simulink model "VS_CS_R4"  (R2018a)
settings: Solver=ode45  StartTime=0.0  StopTime=0.1  FixedStep=50e-6  RelTol=1e-9
libraries: fl_lib x12, nesl_utility x6
settings Model: Creator=mmi-vsa  LastModifiedBy=acs-mmi
settings DataIOCC: SaveFormat=Array
settings OptimizationCC: BlockReduction=off  BooleanDataType=off  LifeSpan=inf
settings DebuggingCC: SaveWithParameterizedLinksMsg=none  UnderspecifiedInitializationDetection=Classic  MergeDetectMultiDrivingBlocksExec=none  SignalResolutionControl=TryResolveAllWithWarning  SFUnexpectedBacktrackingDiag=warning  SFNoUnconditionalDefaultTransitionDiag=warning  SFExecutionAtInitializationDiag=none
settings HardwareCC: ProdBitPerPointer=32  ProdBitPerSizeT=32  ProdBitPerPtrDiffT=32  ProdLargestAtomicFloat=None  ProdIntDivRoundTo=Undefined  ProdEndianess=Unspecified  ProdWordSize=32  ProdHWDeviceType=32-bit Generic  TargetUnknown=on
settings ModelReferenceCC: PropagateSignalLabelsOutOfModel=off
settings CodeAppCC: StateflowObjectComments=on
settings GRTTargetCC: TargetLangStandard=C89/C90 (ANSI)  GeneratePreprocessorConditionals=Disable all
settings ConfigComp: CovMetricSettings=dw  CovHtmlReporting=on  CovSaveCumulativeToWorkspaceVar=on  CovSaveSingleToWorkspaceVar=on  CovExternalEMLEnable=off  CovSFcnEnable=off
settings SimscapeCC: SimscapeNormalizeSystem=off

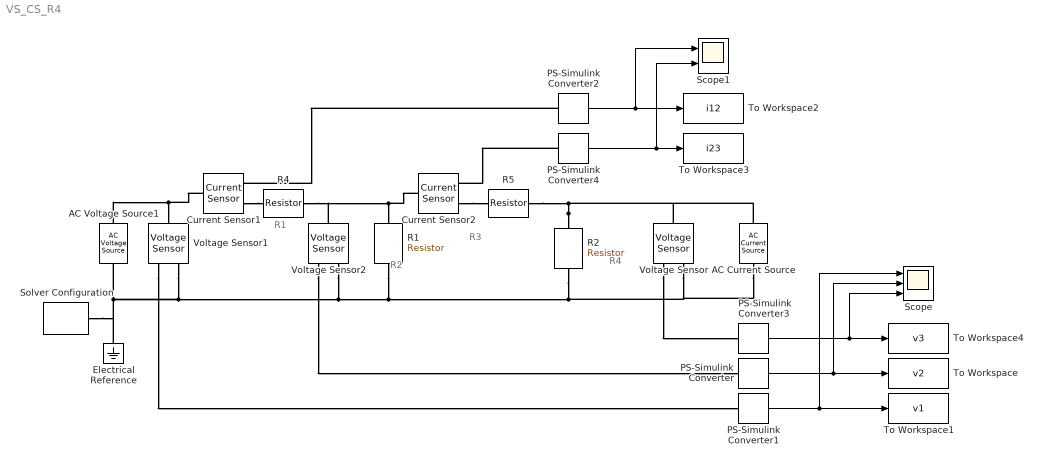
== system VS_CS_R4 ==
  note: R4
  note: R2
  note: R3
  note: R1
  AC Current Source : fl_lib/Electrical/Electrical Sources/AC Current Source  amp=1 A  shift=90 deg  frequency=50 Hz  omega=0 rad/s
      settings: SourceProductName=Simscape  SourceProductBaseCode=SS
  AC Voltage Source1 : fl_lib/Electrical/Electrical Sources/AC Voltage Source  amp=10 V  shift=90 deg  frequency=50 Hz  omega=0 rad/s
  Current Sensor1 : fl_lib/Electrical/Electrical Sensors/Current Sensor
  Current Sensor2 : fl_lib/Electrical/Electrical Sensors/Current Sensor
  Electrical Reference : fl_lib/Electrical/Electrical Elements/Electrical Reference
  PS-Simulink Converter{,1..4} (5 alike) : nesl_utility/PS-Simulink Converter  PhysicalDomain=network_engine_domain  SubClassName=ps_output  LeftPortType=input  RightPortType=output  PseudoPeriodic=off  Frequencies=[]  Unit=1  AffineConversion=off
  R1 : fl_lib/Electrical/Electrical Elements/Resistor  R=1 Ohm  i_specify=off  i_priority=High  i=0 A  i_nominal_specify=off  i_nominal_unit=A  i_nominal_value=1  v_specify=off  v_priority=High  v=0 V  v_nominal_specify=off  v_nominal_unit=V  v_nominal_value=1
  R2 : fl_lib/Electrical/Electrical Elements/Resistor  R=5 Ohm  i_specify=off  i_priority=High  i=0 A  i_nominal_specify=off  i_nominal_unit=A  i_nominal_value=1  v_specify=off  v_priority=High  v=0 V  v_nominal_specify=off  v_nominal_unit=V  v_nominal_value=1
  R4 : fl_lib/Electrical/Electrical Elements/Resistor  R=1 Ohm  i_specify=off  i_priority=High  i=0 A  i_nominal_specify=off  i_nominal_unit=A  i_nominal_value=1  v_specify=off  v_priority=High  v=0 V  v_nominal_specify=off  v_nominal_unit=V  v_nominal_value=1
  R5 : fl_lib/Electrical/Electrical Elements/Resistor  R=10 Ohm  i_specify=off  i_priority=High  i=0 A  i_nominal_specify=off  i_nominal_unit=A  i_nominal_value=1  v_specify=off  v_priority=High  v=0 V  v_nominal_specify=off  v_nominal_unit=V  v_nominal_value=1
  Scope : Scope  NumInputPorts=3
  Scope1 : Scope  NumInputPorts=2
  Solver Configuration : nesl_utility/Solver Configuration  PhysicalDomain=network_engine_domain  SubClassName=solver  LeftPortType=input  RightPortType=generic  Tones=[]  Harmonics=[]  SimulateNoise=off  Profile=off  UseLocalSampling=off  EnableSwitchedLinearOptims=on  FrequencyDomain=off  UseCCode=off  RelTol=0.001  AbsTol=1e-06  MinStep=1e-09  ToWorkspace=off  RevertToSquareIcSolve=off  NumHomotopyIterations=100  PhasorMode=off  PhasorModeNumHarmonics=1  DoDC=off  ResidualTolerance=1e-09  UseLocalSolver=on  LocalSolverChoice=NE_TRAPEZOIDAL_ADVANCER  LocalSolverSampleTime=0.0001  DoFixedCost=on  MaxNonlinIter=3  MaxModeIter=2  LinearAlgebra=Sparse  EquationFormulation=NE_TIME_EF  DelaysMemoryBudget=1024  AutomaticFiltering=on  FilteringTimeConstant=0.001
  To Workspace : ToWorkspace  VariableName=v2  SampleTime=-1
  To Workspace1 : ToWorkspace  VariableName=v1  SampleTime=-1
  To Workspace2 : ToWorkspace  VariableName=i12  SampleTime=-1
  To Workspace3 : ToWorkspace  VariableName=i23  SampleTime=-1
  To Workspace4 : ToWorkspace  VariableName=v3  SampleTime=-1
  Voltage Sensor : fl_lib/Electrical/Electrical Sensors/Voltage Sensor
  Voltage Sensor1 : fl_lib/Electrical/Electrical Sensors/Voltage Sensor
  Voltage Sensor2 : fl_lib/Electrical/Electrical Sensors/Voltage Sensor
  wires:
  PS-Simulink Converter/1 -> Scope/2, To Workspace/1
  PS-Simulink Converter1/1 -> Scope/1, To Workspace1/1
  PS-Simulink Converter2/1 -> Scope1/1, To Workspace2/1
  PS-Simulink Converter3/1 -> Scope/3, To Workspace4/1
  PS-Simulink Converter4/1 -> Scope1/2, To Workspace3/1
  connections:
  Voltage Sensor2/LConn1 -- R4/LConn1 -- Current Sensor2/LConn1 -- R1/LConn1
  R2/LConn1 -- AC Current Source/LConn1 -- Voltage Sensor/LConn1 -- R5/LConn1
  PS-Simulink Converter2/LConn1 -- Current Sensor1/RConn1
  R1/RConn1 -- Electrical Reference/LConn1 -- Solver Configuration/RConn1 -- AC Voltage Source1/RConn1 -- Voltage Sensor1/RConn2 -- Voltage Sensor2/RConn2 -- AC Current Source/RConn1 -- Voltage Sensor/RConn2 -- R2/RConn1
  Voltage Sensor1/RConn1 -- PS-Simulink Converter1/LConn1
  Voltage Sensor2/RConn1 -- PS-Simulink Converter/LConn1
  Voltage Sensor/RConn1 -- PS-Simulink Converter3/LConn1
  AC Voltage Source1/LConn1 -- Current Sensor1/LConn1 -- Voltage Sensor1/LConn1
  Current Sensor1/RConn2 -- R4/RConn1
  Current Sensor2/RConn2 -- R5/RConn1
  PS-Simulink Converter4/LConn1 -- Current Sensor2/RConn1
